simulink model "lab3"  (R2018b)
settings: Solver=ode4  StartTime=0.0  StopTime=10.0  FixedStep=0.01  RelTol=1e-3
values from neighbouring files (symbols this model uses):
  Ad1 = double(phi(0.01))    [scriptlab3.m]
  Bd1 = double(integr(0.01))    [scriptlab3.m]
  Cd = C    [scriptlab3.m]
  Dd = D    [scriptlab3.m]
undefined symbols (not defined in the file or in its folder): den1z, den2z, num1z, num2z
settings Model: Creator=grecu  LastModifiedBy=grecu

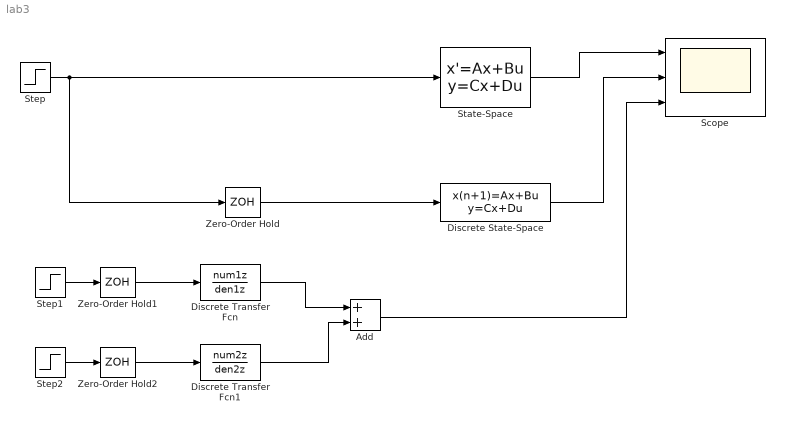
== system lab3 ==
  Add : Sum
  Discrete Transfer Fcn : DiscreteTransferFcn  Numerator=num1z  Denominator=den1z
  Discrete Transfer Fcn1 : DiscreteTransferFcn  Numerator=num2z  Denominator=den2z
  Discrete State-Space : DiscreteStateSpace  A=Ad1  B=Bd1  C=Cd  D=Dd  SampleTime=-1
  Scope : Scope  NumInputPorts=3
  State-Space : StateSpace  A=[-1, 0, 0; -1, -2 ,-101; 1, 1, 0]  B=[0,1;1,-1;0,0]  C=[1,0,101]  D=[0,0]  InitialCondition=0
  Step : Step  After=[1;-2]  SampleTime=0
  Step1 : Step  SampleTime=0
  Step2 : Step  After=-2  SampleTime=0
  Zero-Order Hold : ZeroOrderHold  SampleTime=0.01
  Zero-Order Hold1 : ZeroOrderHold  SampleTime=0.01
  Zero-Order Hold2 : ZeroOrderHold  SampleTime=0.01
  wires:
  Step/1 -> Zero-Order Hold/1, State-Space/1
  State-Space/1 -> Scope/1
  Zero-Order Hold/1 -> Discrete State-Space/1
  Discrete State-Space/1 -> Scope/2
  Discrete Transfer Fcn/1 -> Add/1
  Discrete Transfer Fcn1/1 -> Add/2
  Add/1 -> Scope/3
  Step2/1 -> Zero-Order Hold2/1
  Zero-Order Hold2/1 -> Discrete Transfer Fcn1/1
  Step1/1 -> Zero-Order Hold1/1
  Zero-Order Hold1/1 -> Discrete Transfer Fcn/1
